simulink model "ecart"  (R2020a)
settings: Solver=VariableStepAuto  StartTime=0.0  StopTime=30  RelTol=1e-3
values from neighbouring files (symbols this model uses):
  Af = 1    [FrameVariables.m]
  Bm = (Km*Current_nl)/Omega_nl    (= 0.00282063037873)    [FrameVariables.m]
  Cd = 0.32    [FrameVariables.m]
  D = 1.2    [FrameVariables.m]
  g = 9.8    [FrameVariables.m]
  Gr = 80/11    (= 7.27272727273)    [FrameVariables.m]
  Jm = 4.5*10^-4    (= 0.00045)    [FrameVariables.m]
  Jw = 4    [FrameVariables.m]
  Kb = (T_stall*R)/(Omega_nl*Km)    (= 0.0829409650922)    [FrameVariables.m]
  Km = 0.310    (= 0.31)    [FrameVariables.m]
  L = 0.485*10^-3    (= 0.000485)    [FrameVariables.m]
  M = Mv+Md    (= 180)    [FrameVariables.m]
  R = 0.38    [FrameVariables.m]
  r = 0.2    [FrameVariables.m]
  theta = 0.08    [FrameVariables.m]
  v = 0.2    [FrameVariables.m]
libraries: simulink x1
settings Model: Creator=shasi  LastModifiedBy=shasi

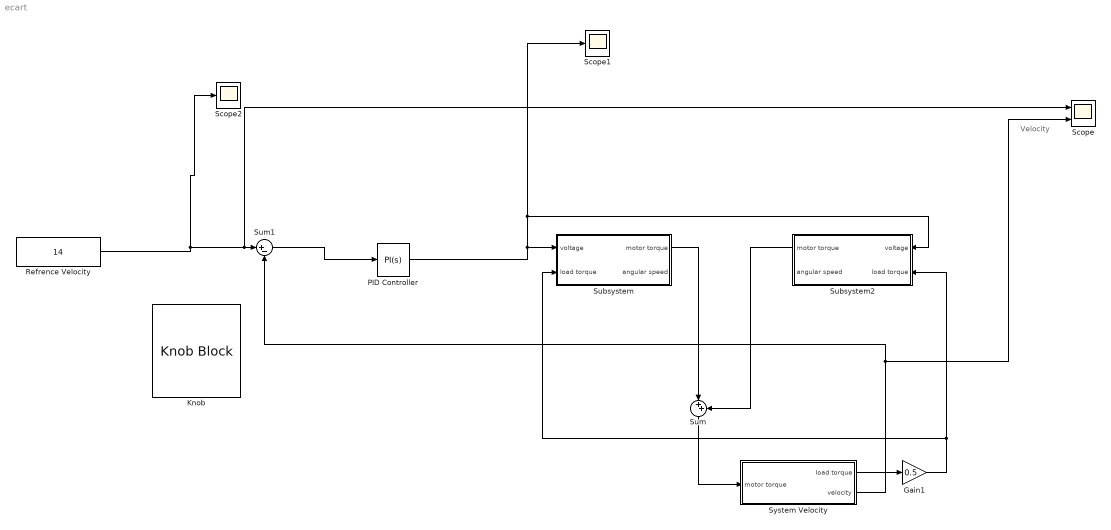
== system ecart ==
  note: Velocity
  Gain1 : Gain  Gain=0.5
  Knob : KnobBlock  ScaleMax=14  TickInterval=1
  PID Controller : simulink/Continuous/PID Controller  Controller=PI  Form=Parallel  TimeDomain=Continuous-time  UseExternalTs=off  SampleTime=-1  IntegratorMethod=Forward Euler  FilterMethod=Forward Euler  ControllerParametersSource=internal  P=2.4  I=0.25  D=5  UseFilter=on  N=0.1  TunerSelectOption=Transfer Function Based (PID Tuner App)  ZeroCross=off  InitialConditionSource=internal  InitialConditionForIntegrator=0  InitialConditionForFilter=0  DifferentiatorICPrevScaledInput=0  ExternalReset=none  IgnoreLimit=on  TrackingMode=off  Kt=10  LimitOutput=on  UpperSaturationLimit=48  LowerSaturationLimit=0  LinearizeAsGain=off  AntiWindupMode=clamping  Kb=1  POutMin=[]  POutMax=[]  IOutMin=[]  IOutMax=[]  DOutMin=[]  DOutMax=[]  NOutMin=[]  NOutMax=[]  SumOutMin=[]  SumOutMax=[]  SaturationOutMin=[]  SaturationOutMax=[]  PParamMin=[]  PParamMax=[]  IParamMin=[]  IParamMax=[]  DParamMin=[]  DParamMax=[]  NParamMin=[]  NParamMax=[]  KbParamMin=[]  KbParamMax=[]  KtParamMin=[]  KtParamMax=[]  KbOutMin=[]  KbOutMax=[]  KtOutMin=[]  KtOutMax=[]  IntegratorOutMin=[]  IntegratorOutMax=[]  FilterOutMin=[]  FilterOutMax=[]  SumI1OutMin=[]  SumI1OutMax=[]  SumI2OutMin=[]  SumI2OutMax=[]  SumI3OutMin=[]  SumI3OutMax=[]  SumI4OutMin=[]  SumI4OutMax=[]  SumDOutMin=[]  SumDOutMax=[]  DifferentiatorOutMin=[]  DifferentiatorOutMax=[]  FilterDiffOutCoefMin=[]  FilterDiffOutCoefMax=[]  ReciprocalOutMin=[]  ReciprocalOutMax=[]  SumDenOutMin=[]  SumDenOutMax=[]  SumNumOutMin=[]  SumNumOutMax=[]  DivideOutMin=[]  DivideOutMax=[]  UdiffTsProdOutMin=[]  UdiffTsProdOutMax=[]  NTsProdOutMin=[]  NTsProdOutMax=[]  UintegralTsProdOutMin=[]  UintegralTsProdOutMax=[]  UngainTsProdOutMin=[]  UngainTsProdOutMax=[]  IntegratorContinuousStateAttributes=''  IntegratorStateMustResolveToSignalObject=off  IntegratorRTWStateStorageClass=Auto  FilterContinuousStateAttributes=''  FilterStateMustResolveToSignalObject=off  FilterRTWStateStorageClass=Auto  ParallelPVariant=InternalParameters  IdealPVariant=Disabled  IVariant=InternalParameters  DVariant=Disabled  IntegratorVariant=Continuous  SatVariant=Enabled  AWVariant=ContClampingParallel  PCopyVariant=Disabled  TRVariant=Disabled  FdbkBlocksVariant=Forward  IdealPFdbkVariant=Disabled  SatFdbkVariant=Disabled  DerivativeFilterVariant=Disabled  NVariant=Disabled  NCopyVariant=Disabled_SignalSpec  FilterICVariant=Disabled  IntegratorICVariant=InternalICs  ExternalResetVariant=Disabled  TRSumVariant=Passthrough  SumFdbkVariant=Disabled  SumVariant=Sum_PI  TsampFilterVariant=InternalTs  TsampNgainVariant=Passthrough  TsampIntegralVariant=Passthrough
  "Refrence Velocity " : Constant  Value=14
  Scope : Scope  NumInputPorts=2
  Scope1 : Scope
  Scope2 : Scope
  Subsystem : Subsystem
  Subsystem2 : Subsystem
  Sum : Sum  Inputs=|++
  Sum1 : Sum  Inputs=|+-
  System Velocity : Subsystem
  wires:
  Subsystem/1(motor torque) -> Sum/1
  Subsystem2/1(motor torque) -> Sum/2
  Sum/1 -> System Velocity/1(motor torque)
  System Velocity/1(load torque) -> Gain1/1
  System Velocity/2(velocity) -> Sum1/2, Scope/2
  Gain1/1 -> Subsystem2/2(load torque), Subsystem/2(load torque)
  "Refrence Velocity "/1 -> Scope2/1, Scope/1, Sum1/1
  PID Controller/1 -> Subsystem/1(voltage), Scope1/1, Subsystem2/1(voltage)
  Sum1/1 -> PID Controller/1

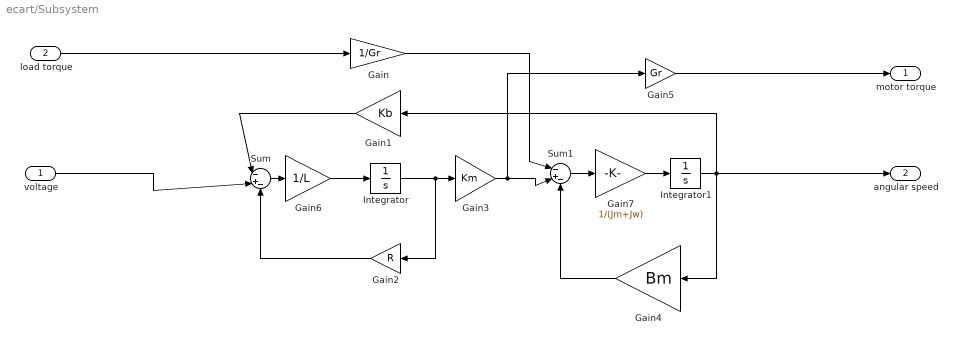
== system ecart/Subsystem ==
  voltage : Inport
  load torque : Inport  Port=2
  Gain : Gain  Gain=1/Gr
  Gain1 : Gain  Gain=Kb
  Gain2 : Gain  Gain=R
  Gain3 : Gain  Gain=Km
  Gain4 : Gain  Gain=Bm
  Gain5 : Gain  Gain=Gr
  Gain6 : Gain  Gain=1/L
  Gain7 : Gain  Gain=1/(Jm+Jw)
  Integrator : Integrator
  Integrator1 : Integrator
  Sum : Sum  Inputs=|-+-
  Sum1 : Sum  Inputs=|-+-
  motor torque : Outport
  angular speed : Outport  Port=2
  wires:
  Gain7/1 -> Integrator1/1
  Gain3/1 -> Gain5/1, Sum1/2
  Integrator1/1 -> Gain1/1, angular speed/1, Gain4/1
  Sum/1 -> Gain6/1
  Gain6/1 -> Integrator/1
  Sum1/1 -> Gain7/1
  Gain2/1 -> Sum/3
  Integrator/1 -> Gain3/1, Gain2/1
  Gain1/1 -> Sum/1
  Gain4/1 -> Sum1/3
  load torque/1 -> Gain/1
  voltage/1 -> Sum/2
  Gain/1 -> Sum1/1
  Gain5/1 -> motor torque/1

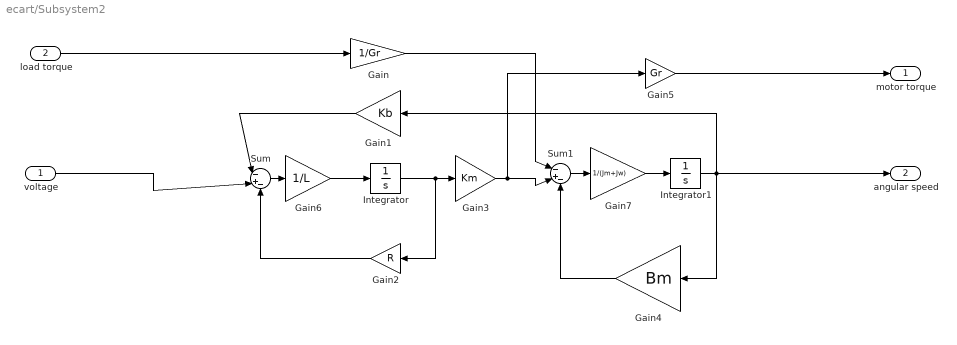
== system ecart/Subsystem2 ==
  voltage : Inport
  load torque : Inport  Port=2
  Gain : Gain  Gain=1/Gr
  Gain1 : Gain  Gain=Kb
  Gain2 : Gain  Gain=R
  Gain3 : Gain  Gain=Km
  Gain4 : Gain  Gain=Bm
  Gain5 : Gain  Gain=Gr
  Gain6 : Gain  Gain=1/L
  Gain7 : Gain  Gain=1/(Jm+Jw)
  Integrator : Integrator
  Integrator1 : Integrator
  Sum : Sum  Inputs=|-+-
  Sum1 : Sum  Inputs=|-+-
  motor torque : Outport
  angular speed : Outport  Port=2
  wires:
  Gain4/1 -> Sum1/3
  Gain5/1 -> motor torque/1
  Gain1/1 -> Sum/1
  Integrator/1 -> Gain2/1, Gain3/1
  Gain/1 -> Sum1/1
  Gain2/1 -> Sum/3
  voltage/1 -> Sum/2
  Sum1/1 -> Gain7/1
  load torque/1 -> Gain/1
  Gain6/1 -> Integrator/1
  Sum/1 -> Gain6/1
  Integrator1/1 -> Gain1/1, Gain4/1, angular speed/1
  Gain3/1 -> Sum1/2, Gain5/1
  Gain7/1 -> Integrator1/1

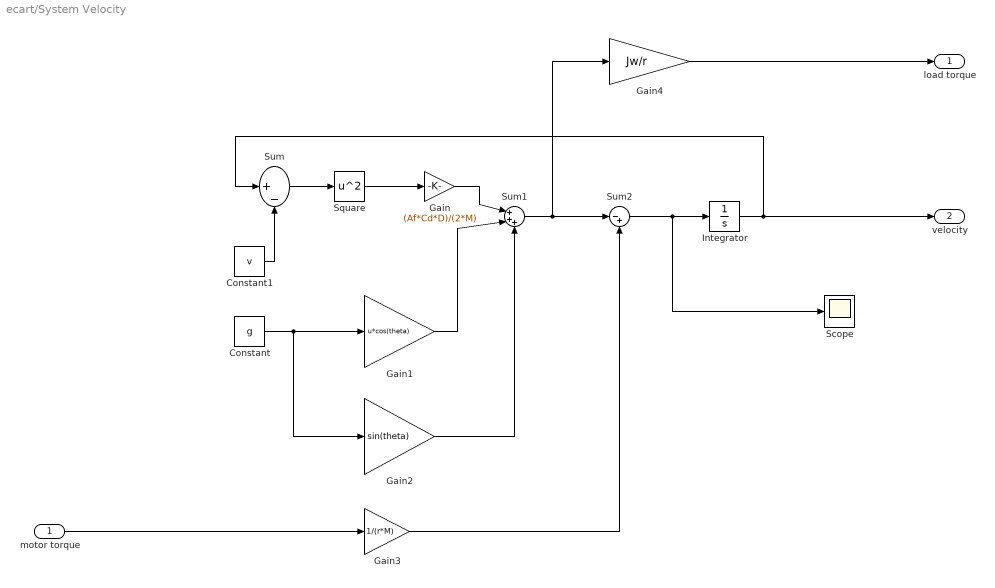
== system ecart/System Velocity ==
  motor torque : Inport
  Constant : Constant  Value=g
  Constant1 : Constant  Value=v
  Gain : Gain  Gain=(Af*Cd*D)/(2*M)
  Gain1 : Gain  Gain=u*cos(theta)
  Gain2 : Gain  Gain=sin(theta)
  Gain3 : Gain  Gain=1/(r*M)
  Gain4 : Gain  Gain=Jw/r
  Integrator : Integrator
  Scope : Scope
  Square : Math  Operator=square  SaturateOnIntegerOverflow=on
  Sum : Sum  Inputs=|+-
  Sum1 : Sum  Inputs=|+++
  Sum2 : Sum  Inputs=|-+
  load torque : Outport
  velocity : Outport  Port=2
  wires:
  Sum1/1 -> Sum2/1, Gain4/1
  Sum2/1 -> Scope/1, Integrator/1
  Constant/1 -> Gain2/1, Gain1/1
  Gain3/1 -> Sum2/2
  Gain1/1 -> Sum1/2
  Gain2/1 -> Sum1/3
  Square/1 -> Gain/1
  Sum/1 -> Square/1
  Constant1/1 -> Sum/2
  motor torque/1 -> Gain3/1
  Gain/1 -> Sum1/1
  Gain4/1 -> load torque/1
  Integrator/1 -> velocity/1, Sum/1
